simulink model "IndustrialMicrogrid"  (R2023a)
settings: Solver=FixedStepDiscrete  StartTime=0.0  StopTime=10  FixedStep=Ts  RelTol=1e-3
PostLoadFcn:
  | IndustrialMicrogridInputData
  | GfmGridFormingConverterInputParameters
model workspace (MAT data in the model file):
  caseNum = 2
undefined symbols (not defined in the file): base, BESS, DiscIntNeverNeededParam, grid, Grid, gridInverter, machine, microgrid, PV, PVInverter, PVTransformer, scrFactorRg, scrFactorXg, transformer, Ts
libraries: ee_lib x112, eeGeneralControl x104, nesl_utility_internal x64, simulink x56, nesl_utility x37, fl_lib x29, slpidlib x13, eeTransforms x11, eeTotalHarmonicDistorsion x8, eeRmsMeasurement x4, eeSinusoidalMeasurement x4, simulink_extras x2
(part 8 of 14)

== system IndustrialMicrogrid/MG2 Primary Substation/Microgrid Controller 2/Planned Island/Control for Zero Powerflow1 ==
  Bus Element In{,1..4} (5 alike) : Inport  PortName=ControlRoom  Element=PlannedIslandCmd2
  In Bus Element7 : Inport  Port=2  PortName=mPCCPLL2  Element=PCC2.mPCC2.activepower
  In Bus Element1 : Inport  Port=2  PortName=mPCCPLL2  Element=PCC2.mPCC2.reactivepower
  Logical Operator : Logic  AllPortsSameDT=off  OutDataTypeStr=boolean
  PID Frequency : slpidlib/PID Controller  Controller=PI  Form=Parallel  TimeDomain=Discrete-time  UseExternalTs=off  SampleTime=2*Ts  IntegratorMethod=Forward Euler  FilterMethod=Forward Euler  ControllerParametersSource=internal  P=KpPPlannedIsland  I=KiPPlannedIsland  UseKiTs=off  D=0  N=100  UseFilter=on  TunerSelectOption=Frequency Response Based  InitialConditionSource=internal  InitialConditionForIntegrator=0  InitialConditionForFilter=0  DifferentiatorICPrevScaledInput=0  ExternalReset=none  TrackingMode=off  Kt=1  LimitOutput=off  SatLimitsSource=internal  UpperSaturationLimit=0.05  LowerSaturationLimit=-0.05  LinearizeAsGain=on  AntiWindupMode=clamping  Kb=1  LimitIntegrator=off  UpperIntegratorSaturationLimit=inf  LowerIntegratorSaturationLimit=-inf  POutMin=[]  POutMax=[]  IOutMin=[]  IOutMax=[]  DOutMin=[]  DOutMax=[]  NOutMin=[]  NOutMax=[]  SumOutMin=[]  SumOutMax=[]  SaturationOutMin=[]  SaturationOutMax=[]  PParamMin=[]  PParamMax=[]  IParamMin=[]  IParamMax=[]  DParamMin=[]  DParamMax=[]  NParamMin=[]  NParamMax=[]  KbParamMin=[]  KbParamMax=[]  KtParamMin=[]  KtParamMax=[]  KbOutMin=[]  KbOutMax=[]  KtOutMin=[]  KtOutMax=[]  IntegratorOutMin=[]  IntegratorOutMax=[]  FilterOutMin=[]  FilterOutMax=[]  SumI1OutMin=[]  SumI1OutMax=[]  SumI2OutMin=[]  SumI2OutMax=[]  SumI3OutMin=[]  SumI3OutMax=[]  SumI4OutMin=[]  SumI4OutMax=[]  SumDOutMin=[]  SumDOutMax=[]  DifferentiatorOutMin=[]  DifferentiatorOutMax=[]  FilterDiffOutCoefMin=[]  FilterDiffOutCoefMax=[]  ReciprocalOutMin=[]  ReciprocalOutMax=[]  SumDenOutMin=[]  SumDenOutMax=[]  SumNumOutMin=[]  SumNumOutMax=[]  DivideOutMin=[]  DivideOutMax=[]  UdiffTsProdOutMin=[]  UdiffTsProdOutMax=[]  NTsProdOutMin=[]  NTsProdOutMax=[]  UintegralTsProdOutMin=[]  UintegralTsProdOutMax=[]  UngainTsProdOutMin=[]  UngainTsProdOutMax=[]  ClampingZeroOutDataTypeStr=Inherit: Inherit via back propagation  ClampingZeroOutMin=[]  ClampingZeroOutMax=[]  FilterDenConstantOutDataTypeStr=Inherit: Inherit via back propagation  FilterDenConstantOutMin=[]  FilterDenConstantOutMax=[]  PCopyOutDataTypeStr=Inherit: Inherit via back propagation  PCopyOutMin=[]  PCopyOutMax=[]  NCopyOutDataTypeStr=Inherit: Inherit via back propagation  NCopyOutMin=[]  NCopyOutMax=[]  IntegratorContinuousStateAttributes=''  IntegratorStateMustResolveToSignalObject=off  IntegratorRTWStateStorageClass=Auto  FilterContinuousStateAttributes=''  FilterStateMustResolveToSignalObject=off  FilterRTWStateStorageClass=Auto  ParallelPVariant=InternalParameters  IdealPVariant=Disabled  IVariant=InternalParameters  DVariant=Disabled  IntegratorVariant=Discrete  SatVariant=Disabled  AWVariant=Passthrough  PCopyVariant=Disabled  TRVariant=Disabled  FdbkBlocksVariant=Forward  IdealPFdbkVariant=Disabled  SatFdbkVariant=Disabled  DerivativeFilterVariant=Disabled  NVariant=Disabled  NCopyVariant=Disabled_SignalSpec  FilterICVariant=Disabled  IntegratorICVariant=InternalICs  ExternalResetVariant=Disabled  TRSumVariant=Passthrough  SumFdbkVariant=Disabled  SumVariant=Sum_PI  TsampFilterVariant=InternalTs  TsampNgainVariant=Passthrough  TsampIntegralVariant=Disabled_SignalSpec  ExternalSaturationOutDataTypeStr=Inherit: Same as second input
  PID voltage : slpidlib/PID Controller  Controller=PI  Form=Parallel  TimeDomain=Discrete-time  UseExternalTs=off  SampleTime=2*Ts  IntegratorMethod=Forward Euler  FilterMethod=Forward Euler  ControllerParametersSource=internal  P=KpQPlannedIsland  I=KiQPlannedIsland  UseKiTs=off  D=0  N=100  UseFilter=on  TunerSelectOption=Frequency Response Based  InitialConditionSource=internal  InitialConditionForIntegrator=0  InitialConditionForFilter=0  DifferentiatorICPrevScaledInput=0  ExternalReset=none  TrackingMode=off  Kt=1  LimitOutput=off  SatLimitsSource=internal  UpperSaturationLimit=0.05  LowerSaturationLimit=-0.05  LinearizeAsGain=on  AntiWindupMode=clamping  Kb=1  LimitIntegrator=off  UpperIntegratorSaturationLimit=inf  LowerIntegratorSaturationLimit=-inf  POutMin=[]  POutMax=[]  IOutMin=[]  IOutMax=[]  DOutMin=[]  DOutMax=[]  NOutMin=[]  NOutMax=[]  SumOutMin=[]  SumOutMax=[]  SaturationOutMin=[]  SaturationOutMax=[]  PParamMin=[]  PParamMax=[]  IParamMin=[]  IParamMax=[]  DParamMin=[]  DParamMax=[]  NParamMin=[]  NParamMax=[]  KbParamMin=[]  KbParamMax=[]  KtParamMin=[]  KtParamMax=[]  KbOutMin=[]  KbOutMax=[]  KtOutMin=[]  KtOutMax=[]  IntegratorOutMin=[]  IntegratorOutMax=[]  FilterOutMin=[]  FilterOutMax=[]  SumI1OutMin=[]  SumI1OutMax=[]  SumI2OutMin=[]  SumI2OutMax=[]  SumI3OutMin=[]  SumI3OutMax=[]  SumI4OutMin=[]  SumI4OutMax=[]  SumDOutMin=[]  SumDOutMax=[]  DifferentiatorOutMin=[]  DifferentiatorOutMax=[]  FilterDiffOutCoefMin=[]  FilterDiffOutCoefMax=[]  ReciprocalOutMin=[]  ReciprocalOutMax=[]  SumDenOutMin=[]  SumDenOutMax=[]  SumNumOutMin=[]  SumNumOutMax=[]  DivideOutMin=[]  DivideOutMax=[]  UdiffTsProdOutMin=[]  UdiffTsProdOutMax=[]  NTsProdOutMin=[]  NTsProdOutMax=[]  UintegralTsProdOutMin=[]  UintegralTsProdOutMax=[]  UngainTsProdOutMin=[]  UngainTsProdOutMax=[]  ClampingZeroOutDataTypeStr=Inherit: Inherit via back propagation  ClampingZeroOutMin=[]  ClampingZeroOutMax=[]  FilterDenConstantOutDataTypeStr=Inherit: Inherit via back propagation  FilterDenConstantOutMin=[]  FilterDenConstantOutMax=[]  PCopyOutDataTypeStr=Inherit: Inherit via back propagation  PCopyOutMin=[]  PCopyOutMax=[]  NCopyOutDataTypeStr=Inherit: Inherit via back propagation  NCopyOutMin=[]  NCopyOutMax=[]  IntegratorContinuousStateAttributes=''  IntegratorStateMustResolveToSignalObject=off  IntegratorRTWStateStorageClass=Auto  FilterContinuousStateAttributes=''  FilterStateMustResolveToSignalObject=off  FilterRTWStateStorageClass=Auto  ParallelPVariant=InternalParameters  IdealPVariant=Disabled  IVariant=InternalParameters  DVariant=Disabled  IntegratorVariant=Discrete  SatVariant=Disabled  AWVariant=Passthrough  PCopyVariant=Disabled  TRVariant=Disabled  FdbkBlocksVariant=Forward  IdealPFdbkVariant=Disabled  SatFdbkVariant=Disabled  DerivativeFilterVariant=Disabled  NVariant=Disabled  NCopyVariant=Disabled_SignalSpec  FilterICVariant=Disabled  IntegratorICVariant=InternalICs  ExternalResetVariant=Disabled  TRSumVariant=Passthrough  SumFdbkVariant=Disabled  SumVariant=Sum_PI  TsampFilterVariant=InternalTs  TsampNgainVariant=Passthrough  TsampIntegralVariant=Disabled_SignalSpec  ExternalSaturationOutDataTypeStr=Inherit: Same as second input
  Planned Island Time Delay : Subsystem
  Product{,1..3} (4 alike) : Product
  Subsystem : Subsystem
  Subsystem1 : Subsystem
  Bus Element Out : Outport  PortName=MGController2  Element=plannedisland
  Bus Element Out1 : Outport  PortName=MGController2  Element=plannedislandP
  Bus Element Out2 : Outport  PortName=MGController2  Element=plannedislandQ
  Bus Element Out4 : Outport  PortName=MGController2  Element=activepowererror
  Bus Element Out6 : Outport  PortName=MGController2  Element=reactivepowerrror
  wires:
  Logical Operator/1 -> Planned Island Time Delay/1(In1)
  Planned Island Time Delay/1(MGController) -> Bus Element Out/1
  Bus Element In3/1 -> Planned Island Time Delay/2(In2)
  PID voltage/1 -> Bus Element Out2/1  "REACTIVE POWER"
  Bus Element In2/1 -> Product2/2
  Bus Element In/1 -> Product1/2
  Product2/1 -> Subsystem1/1(REACTIVEPOWER ERROR), PID voltage/1, Bus Element Out6/1  "REACTIVEPOWER ERROR"
  Product1/1 -> PID Frequency/1, Bus Element Out4/1, Subsystem/1(AVTIVE POWER ERROR)  "AVTIVE POWER ERROR"
  PID Frequency/1 -> Bus Element Out1/1  "ACTIVE POWER"
  In Bus Element1/1 -> Product2/1
  In Bus Element7/1 -> Product1/1
  Bus Element In1/1 -> Product/1
  Product/1 -> Logical Operator/1
  Product3/1 -> Logical Operator/2
  Bus Element In4/1 -> Product3/1
  Subsystem/1(Out1) -> Product/2
  Subsystem1/1(Out1) -> Product3/2

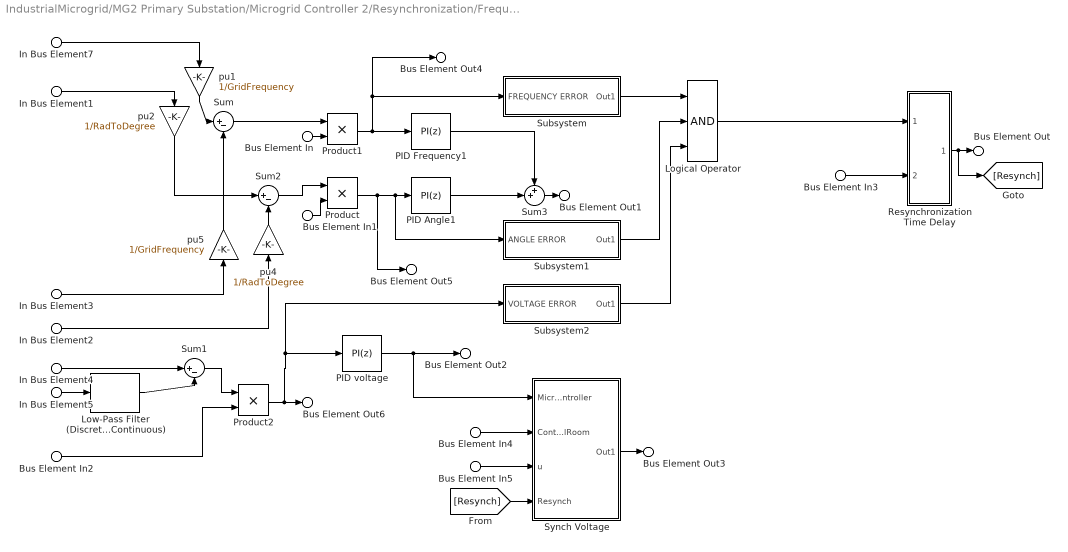
== system IndustrialMicrogrid/MG2 Primary Substation/Microgrid Controller 2/Resynchronization/Frequency and voltage matching ==
  Bus Element In5 : Inport  PortName=BESS2  Element=reactive power
  Bus Element In{,1..4} (5 alike) : Inport  Port=2  PortName=ControlRoom  Element=ResynchCmd2
  In Bus Element7 : Inport  Port=3  PortName=mPCCPLL2  Element=Grid2.frequency
  In Bus Element1 : Inport  Port=3  PortName=mPCCPLL2  Element=Grid2.angle
  In Bus Element4 : Inport  Port=3  PortName=mPCCPLL2  Element=Grid2.voltage
  In Bus Element3 : Inport  Port=3  PortName=mPCCPLL2  Element=Island2.frequency
  In Bus Element2 : Inport  Port=3  PortName=mPCCPLL2  Element=Island2.angle
  In Bus Element5 : Inport  Port=3  PortName=mPCCPLL2  Element=Island2.voltage
  Logical Operator : Logic  Inputs=3  AllPortsSameDT=off  OutDataTypeStr=boolean
  Low-Pass Filter (Discrete or Continuous) : eeGeneralControl/Low-Pass Filter (Discrete or Continuous)  K=1  T=0.04  B=inf  A=-inf  init_option=Inherited from block input  x0=0  Ts=-1
  PID Angle1 : slpidlib/PID Controller  Controller=PI  Form=Parallel  TimeDomain=Discrete-time  UseExternalTs=off  SampleTime=2*Ts  IntegratorMethod=Forward Euler  FilterMethod=Forward Euler  ControllerParametersSource=internal  P=KpAngResynch  I=KiAngResynch  UseKiTs=off  D=0  N=100  UseFilter=on  TunerSelectOption=Frequency Response Based  InitialConditionSource=internal  InitialConditionForIntegrator=0  InitialConditionForFilter=0  DifferentiatorICPrevScaledInput=0  ExternalReset=none  TrackingMode=off  Kt=1  LimitOutput=off  SatLimitsSource=internal  UpperSaturationLimit=0.05  LowerSaturationLimit=-0.05  LinearizeAsGain=on  AntiWindupMode=clamping  Kb=1  LimitIntegrator=off  UpperIntegratorSaturationLimit=inf  LowerIntegratorSaturationLimit=-inf  POutMin=[]  POutMax=[]  IOutMin=[]  IOutMax=[]  DOutMin=[]  DOutMax=[]  NOutMin=[]  NOutMax=[]  SumOutMin=[]  SumOutMax=[]  SaturationOutMin=[]  SaturationOutMax=[]  PParamMin=[]  PParamMax=[]  IParamMin=[]  IParamMax=[]  DParamMin=[]  DParamMax=[]  NParamMin=[]  NParamMax=[]  KbParamMin=[]  KbParamMax=[]  KtParamMin=[]  KtParamMax=[]  KbOutMin=[]  KbOutMax=[]  KtOutMin=[]  KtOutMax=[]  IntegratorOutMin=[]  IntegratorOutMax=[]  FilterOutMin=[]  FilterOutMax=[]  SumI1OutMin=[]  SumI1OutMax=[]  SumI2OutMin=[]  SumI2OutMax=[]  SumI3OutMin=[]  SumI3OutMax=[]  SumI4OutMin=[]  SumI4OutMax=[]  SumDOutMin=[]  SumDOutMax=[]  DifferentiatorOutMin=[]  DifferentiatorOutMax=[]  FilterDiffOutCoefMin=[]  FilterDiffOutCoefMax=[]  ReciprocalOutMin=[]  ReciprocalOutMax=[]  SumDenOutMin=[]  SumDenOutMax=[]  SumNumOutMin=[]  SumNumOutMax=[]  DivideOutMin=[]  DivideOutMax=[]  UdiffTsProdOutMin=[]  UdiffTsProdOutMax=[]  NTsProdOutMin=[]  NTsProdOutMax=[]  UintegralTsProdOutMin=[]  UintegralTsProdOutMax=[]  UngainTsProdOutMin=[]  UngainTsProdOutMax=[]  ClampingZeroOutDataTypeStr=Inherit: Inherit via back propagation  ClampingZeroOutMin=[]  ClampingZeroOutMax=[]  FilterDenConstantOutDataTypeStr=Inherit: Inherit via back propagation  FilterDenConstantOutMin=[]  FilterDenConstantOutMax=[]  PCopyOutDataTypeStr=Inherit: Inherit via back propagation  PCopyOutMin=[]  PCopyOutMax=[]  NCopyOutDataTypeStr=Inherit: Inherit via back propagation  NCopyOutMin=[]  NCopyOutMax=[]  IntegratorContinuousStateAttributes=''  IntegratorStateMustResolveToSignalObject=off  IntegratorRTWStateStorageClass=Auto  FilterContinuousStateAttributes=''  FilterStateMustResolveToSignalObject=off  FilterRTWStateStorageClass=Auto  ParallelPVariant=InternalParameters  IdealPVariant=Disabled  IVariant=InternalParameters  DVariant=Disabled  IntegratorVariant=Discrete  SatVariant=Disabled  AWVariant=Passthrough  PCopyVariant=Disabled  TRVariant=Disabled  FdbkBlocksVariant=Forward  IdealPFdbkVariant=Disabled  SatFdbkVariant=Disabled  DerivativeFilterVariant=Disabled  NVariant=Disabled  NCopyVariant=Disabled_SignalSpec  FilterICVariant=Disabled  IntegratorICVariant=InternalICs  ExternalResetVariant=Disabled  TRSumVariant=Passthrough  SumFdbkVariant=Disabled  SumVariant=Sum_PI  TsampFilterVariant=InternalTs  TsampNgainVariant=Passthrough  TsampIntegralVariant=Disabled_SignalSpec  ExternalSaturationOutDataTypeStr=Inherit: Same as second input
  PID Frequency1 : slpidlib/PID Controller  Controller=PI  Form=Parallel  TimeDomain=Discrete-time  UseExternalTs=off  SampleTime=2*Ts  IntegratorMethod=Forward Euler  FilterMethod=Forward Euler  ControllerParametersSource=internal  P=KpFreResynch  I=KiFreResynch  UseKiTs=off  D=0  N=100  UseFilter=on  TunerSelectOption=Frequency Response Based  InitialConditionSource=internal  InitialConditionForIntegrator=0  InitialConditionForFilter=0  DifferentiatorICPrevScaledInput=0  ExternalReset=none  TrackingMode=off  Kt=1  LimitOutput=off  SatLimitsSource=internal  UpperSaturationLimit=0.05  LowerSaturationLimit=-0.05  LinearizeAsGain=on  AntiWindupMode=clamping  Kb=1  LimitIntegrator=off  UpperIntegratorSaturationLimit=inf  LowerIntegratorSaturationLimit=-inf  POutMin=[]  POutMax=[]  IOutMin=[]  IOutMax=[]  DOutMin=[]  DOutMax=[]  NOutMin=[]  NOutMax=[]  SumOutMin=[]  SumOutMax=[]  SaturationOutMin=[]  SaturationOutMax=[]  PParamMin=[]  PParamMax=[]  IParamMin=[]  IParamMax=[]  DParamMin=[]  DParamMax=[]  NParamMin=[]  NParamMax=[]  KbParamMin=[]  KbParamMax=[]  KtParamMin=[]  KtParamMax=[]  KbOutMin=[]  KbOutMax=[]  KtOutMin=[]  KtOutMax=[]  IntegratorOutMin=[]  IntegratorOutMax=[]  FilterOutMin=[]  FilterOutMax=[]  SumI1OutMin=[]  SumI1OutMax=[]  SumI2OutMin=[]  SumI2OutMax=[]  SumI3OutMin=[]  SumI3OutMax=[]  SumI4OutMin=[]  SumI4OutMax=[]  SumDOutMin=[]  SumDOutMax=[]  DifferentiatorOutMin=[]  DifferentiatorOutMax=[]  FilterDiffOutCoefMin=[]  FilterDiffOutCoefMax=[]  ReciprocalOutMin=[]  ReciprocalOutMax=[]  SumDenOutMin=[]  SumDenOutMax=[]  SumNumOutMin=[]  SumNumOutMax=[]  DivideOutMin=[]  DivideOutMax=[]  UdiffTsProdOutMin=[]  UdiffTsProdOutMax=[]  NTsProdOutMin=[]  NTsProdOutMax=[]  UintegralTsProdOutMin=[]  UintegralTsProdOutMax=[]  UngainTsProdOutMin=[]  UngainTsProdOutMax=[]  ClampingZeroOutDataTypeStr=Inherit: Inherit via back propagation  ClampingZeroOutMin=[]  ClampingZeroOutMax=[]  FilterDenConstantOutDataTypeStr=Inherit: Inherit via back propagation  FilterDenConstantOutMin=[]  FilterDenConstantOutMax=[]  PCopyOutDataTypeStr=Inherit: Inherit via back propagation  PCopyOutMin=[]  PCopyOutMax=[]  NCopyOutDataTypeStr=Inherit: Inherit via back propagation  NCopyOutMin=[]  NCopyOutMax=[]  IntegratorContinuousStateAttributes=''  IntegratorStateMustResolveToSignalObject=off  IntegratorRTWStateStorageClass=Auto  FilterContinuousStateAttributes=''  FilterStateMustResolveToSignalObject=off  FilterRTWStateStorageClass=Auto  ParallelPVariant=InternalParameters  IdealPVariant=Disabled  IVariant=InternalParameters  DVariant=Disabled  IntegratorVariant=Discrete  SatVariant=Disabled  AWVariant=Passthrough  PCopyVariant=Disabled  TRVariant=Disabled  FdbkBlocksVariant=Forward  IdealPFdbkVariant=Disabled  SatFdbkVariant=Disabled  DerivativeFilterVariant=Disabled  NVariant=Disabled  NCopyVariant=Disabled_SignalSpec  FilterICVariant=Disabled  IntegratorICVariant=InternalICs  ExternalResetVariant=Disabled  TRSumVariant=Passthrough  SumFdbkVariant=Disabled  SumVariant=Sum_PI  TsampFilterVariant=InternalTs  TsampNgainVariant=Passthrough  TsampIntegralVariant=Disabled_SignalSpec  ExternalSaturationOutDataTypeStr=Inherit: Same as second input
  PID voltage : slpidlib/PID Controller  Controller=PI  Form=Parallel  TimeDomain=Discrete-time  UseExternalTs=off  SampleTime=2*Ts  IntegratorMethod=Forward Euler  FilterMethod=Forward Euler  ControllerParametersSource=internal  P=KpVolResynch  I=KiVolResynch  UseKiTs=off  D=0  N=100  UseFilter=on  TunerSelectOption=Frequency Response Based  InitialConditionSource=internal  InitialConditionForIntegrator=1  InitialConditionForFilter=0  DifferentiatorICPrevScaledInput=0  ExternalReset=none  TrackingMode=off  Kt=1  LimitOutput=off  SatLimitsSource=internal  UpperSaturationLimit=0.05  LowerSaturationLimit=-0.05  LinearizeAsGain=on  AntiWindupMode=clamping  Kb=1  LimitIntegrator=off  UpperIntegratorSaturationLimit=inf  LowerIntegratorSaturationLimit=-inf  POutMin=[]  POutMax=[]  IOutMin=[]  IOutMax=[]  DOutMin=[]  DOutMax=[]  NOutMin=[]  NOutMax=[]  SumOutMin=[]  SumOutMax=[]  SaturationOutMin=[]  SaturationOutMax=[]  PParamMin=[]  PParamMax=[]  IParamMin=[]  IParamMax=[]  DParamMin=[]  DParamMax=[]  NParamMin=[]  NParamMax=[]  KbParamMin=[]  KbParamMax=[]  KtParamMin=[]  KtParamMax=[]  KbOutMin=[]  KbOutMax=[]  KtOutMin=[]  KtOutMax=[]  IntegratorOutMin=[]  IntegratorOutMax=[]  FilterOutMin=[]  FilterOutMax=[]  SumI1OutMin=[]  SumI1OutMax=[]  SumI2OutMin=[]  SumI2OutMax=[]  SumI3OutMin=[]  SumI3OutMax=[]  SumI4OutMin=[]  SumI4OutMax=[]  SumDOutMin=[]  SumDOutMax=[]  DifferentiatorOutMin=[]  DifferentiatorOutMax=[]  FilterDiffOutCoefMin=[]  FilterDiffOutCoefMax=[]  ReciprocalOutMin=[]  ReciprocalOutMax=[]  SumDenOutMin=[]  SumDenOutMax=[]  SumNumOutMin=[]  SumNumOutMax=[]  DivideOutMin=[]  DivideOutMax=[]  UdiffTsProdOutMin=[]  UdiffTsProdOutMax=[]  NTsProdOutMin=[]  NTsProdOutMax=[]  UintegralTsProdOutMin=[]  UintegralTsProdOutMax=[]  UngainTsProdOutMin=[]  UngainTsProdOutMax=[]  ClampingZeroOutDataTypeStr=Inherit: Inherit via back propagation  ClampingZeroOutMin=[]  ClampingZeroOutMax=[]  FilterDenConstantOutDataTypeStr=Inherit: Inherit via back propagation  FilterDenConstantOutMin=[]  FilterDenConstantOutMax=[]  PCopyOutDataTypeStr=Inherit: Inherit via back propagation  PCopyOutMin=[]  PCopyOutMax=[]  NCopyOutDataTypeStr=Inherit: Inherit via back propagation  NCopyOutMin=[]  NCopyOutMax=[]  IntegratorContinuousStateAttributes=''  IntegratorStateMustResolveToSignalObject=off  IntegratorRTWStateStorageClass=Auto  FilterContinuousStateAttributes=''  FilterStateMustResolveToSignalObject=off  FilterRTWStateStorageClass=Auto  ParallelPVariant=InternalParameters  IdealPVariant=Disabled  IVariant=InternalParameters  DVariant=Disabled  IntegratorVariant=Discrete  SatVariant=Disabled  AWVariant=Passthrough  PCopyVariant=Disabled  TRVariant=Disabled  FdbkBlocksVariant=Forward  IdealPFdbkVariant=Disabled  SatFdbkVariant=Disabled  DerivativeFilterVariant=Disabled  NVariant=Disabled  NCopyVariant=Disabled_SignalSpec  FilterICVariant=Disabled  IntegratorICVariant=InternalICs  ExternalResetVariant=Disabled  TRSumVariant=Passthrough  SumFdbkVariant=Disabled  SumVariant=Sum_PI  TsampFilterVariant=InternalTs  TsampNgainVariant=Passthrough  TsampIntegralVariant=Disabled_SignalSpec  ExternalSaturationOutDataTypeStr=Inherit: Same as second input
  Product : Product
  Product1 : Product
  Product2 : Product
  Resynchronization Time Delay : Subsystem
  Subsystem : Subsystem
  Subsystem1 : Subsystem
  Subsystem2 : Subsystem
  Sum : Sum  Inputs=|+-
  Sum1 : Sum  Inputs=|+-
  Sum2 : Sum  Inputs=|+-
  Sum3 : Sum  Inputs=++|
  Synch Voltage : Subsystem
  pu1 : Gain  Gain=1/GridFrequency
  pu2 : Gain  Gain=1/RadToDegree
  pu4 : Gain  Gain=1/RadToDegree
  pu5 : Gain  Gain=1/GridFrequency
  Bus Element Out : Outport  PortName=MGController2  Element=resynch
  Bus Element Out1 : Outport  PortName=MGController2  Element=synchfrequency
  Bus Element Out2 : Outport  PortName=MGController2  Element=synchvoltage
  Bus Element Out3 : Outport  PortName=MGController2  Element=synchvoltagedpr
  Bus Element Out4 : Outport  PortName=MGController2  Element=frequencyerror
  Bus Element Out5 : Outport  PortName=MGController2  Element=phaseerror
  Bus Element Out6 : Outport  PortName=MGController2  Element=voltagemagerror
  wires:
  Sum/1 -> Product1/1
  pu1/1 -> Sum/1
  pu4/1 -> Sum2/2
  pu2/1 -> Sum2/1
  pu5/1 -> Sum/2
  In Bus Element2/1 -> pu4/1
  In Bus Element3/1 -> pu5/1
  Sum1/1 -> Product2/1
  Subsystem/1(Out1) -> Logical Operator/1
  Subsystem1/1(Out1) -> Logical Operator/2
  Subsystem2/1(Out1) -> Logical Operator/3
  Sum3/1 -> Bus Element Out1/1
  PID Frequency1/1 -> Sum3/1
  PID Angle1/1 -> Sum3/2
  Sum2/1 -> Product/1
  Product/1 -> Bus Element Out5/1, Subsystem1/1(ANGLE ERROR), PID Angle1/1
  Product1/1 -> Bus Element Out4/1, Subsystem/1(FREQUENCY ERROR), PID Frequency1/1
  Product2/1 -> Subsystem2/1(VOLTAGE ERROR), PID voltage/1, Bus Element Out6/1
  Bus Element In/1 -> Product1/2
  Bus Element In1/1 -> Product/2
  Bus Element In2/1 -> Product2/2
  In Bus Element7/1 -> pu1/1
  In Bus Element1/1 -> pu2/1
  In Bus Element4/1 -> Sum1/1
  In Bus Element5/1 -> Low-Pass Filter (Discrete or Continuous)/1
  PID voltage/1 -> Bus Element Out2/1, Synch Voltage/1(MicrogridController)
  Bus Element In3/1 -> Resynchronization Time Delay/2(In2)
  Resynchronization Time Delay/1(MGController) -> [Resynch], Bus Element Out/1
  Logical Operator/1 -> Resynchronization Time Delay/1(In1)
  Bus Element In4/1 -> Synch Voltage/2(ControlRoom)
  Bus Element In5/1 -> Synch Voltage/3(u)
  Synch Voltage/1(Out1) -> Bus Element Out3/1
  [Resynch] -> Synch Voltage/4(Resynch)
  Low-Pass Filter (Discrete or Continuous)/1 -> Sum1/2

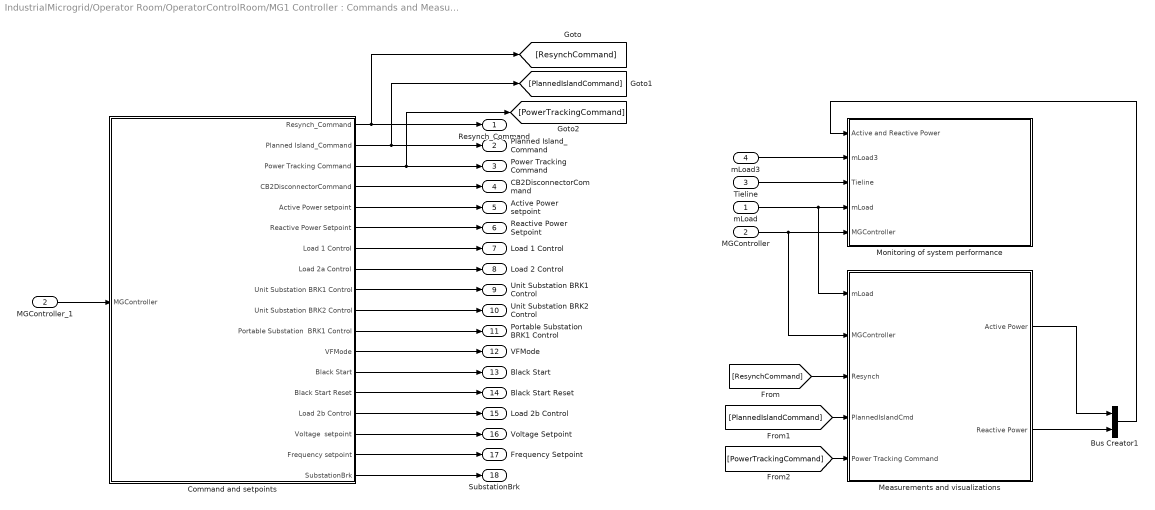
== system IndustrialMicrogrid/Operator Room/OperatorControlRoom/MG1 Controller : Commands and Measurements/Microgrid Controller 1 : Commands and Measurements ==
  mLoad : Inport
  MGController : Inport  Port=2
  Tieline : Inport  Port=3
  mLoad3 : Inport  Port=4
  Bus Creator1 : BusCreator  Inputs=2
  Command and setpoints : Subsystem
  MGController_1 : InportShadow  Port=2
  "Measurements and visualizations " : Subsystem
  Monitoring of system performance : Subsystem
  Resynch_Command : Outport
  Planned Island_Command : Outport  Port=2
  Power Tracking Command : Outport  Port=3
  CB2DisconnectorCommand : Outport  Port=4
  Active Power setpoint : Outport  Port=5
  Reactive Power Setpoint : Outport  Port=6
  Load 1 Control : Outport  Port=7
  Load 2 Control : Outport  Port=8
  Unit Substation BRK1 Control : Outport  Port=9
  Unit Substation BRK2 Control : Outport  Port=10
  Portable Substation  BRK1 Control : Outport  Port=11
  VFMode : Outport  Port=12
  Black Start : Outport  Port=13
  Black Start Reset : Outport  Port=14
  Load 2b Control : Outport  Port=15
  Voltage Setpoint : Outport  Port=16
  Frequency Setpoint : Outport  Port=17
  SubstationBrk : Outport  Port=18
  wires:
  mLoad/1 -> "Measurements and visualizations "/1(mLoad), Monitoring of system performance/4(mLoad)
  [PlannedIslandCommand] -> "Measurements and visualizations "/4(PlannedIslandCmd)
  Command and setpoints/2(Planned Island_Command) -> Planned Island_Command/1, [PlannedIslandCommand]
  Command and setpoints/3(Power Tracking Command) -> Power Tracking Command/1, [PowerTrackingCommand]
  Command and setpoints/1(Resynch_Command) -> Resynch_Command/1, [ResynchCommand]
  Command and setpoints/4(CB2DisconnectorCommand) -> CB2DisconnectorCommand/1
  MGController/1 -> "Measurements and visualizations "/2(MGController), Monitoring of system performance/5(MGController)
  MGController_1/1 -> Command and setpoints/1(MGController)
  [ResynchCommand] -> "Measurements and visualizations "/3(Resynch)
  [PowerTrackingCommand] -> "Measurements and visualizations "/5(Power Tracking Command)
  Command and setpoints/5(Active Power setpoint) -> Active Power setpoint/1
  Command and setpoints/6(Reactive Power Setpoint) -> Reactive Power Setpoint/1
  Command and setpoints/10(Unit Substation BRK2 Control) -> Unit Substation BRK2 Control/1
  Command and setpoints/8(Load 2a Control) -> Load 2 Control/1
  Command and setpoints/9(Unit Substation BRK1 Control) -> Unit Substation BRK1 Control/1
  Command and setpoints/7(Load 1 Control) -> Load 1 Control/1
  Command and setpoints/11(Portable Substation  BRK1 Control) -> Portable Substation  BRK1 Control/1
  Command and setpoints/12(VFMode) -> VFMode/1
  Command and setpoints/14(Black Start Reset) -> Black Start Reset/1
  Command and setpoints/13(Black Start) -> Black Start/1
  Command and setpoints/15(Load 2b Control) -> Load 2b Control/1
  Command and setpoints/16(Voltage  setpoint) -> Voltage Setpoint/1
  Command and setpoints/17(Frequency setpoint) -> Frequency Setpoint/1
  Command and setpoints/18(SubstationBrk) -> SubstationBrk/1
  "Measurements and visualizations "/2(Reactive Power) -> Bus Creator1/2
  "Measurements and visualizations "/1(Active Power) -> Bus Creator1/1
  Bus Creator1/1 -> Monitoring of system performance/1(Active and Reactive Power)
  Tieline/1 -> Monitoring of system performance/3(Tieline)
  mLoad3/1 -> Monitoring of system performance/2(mLoad3)

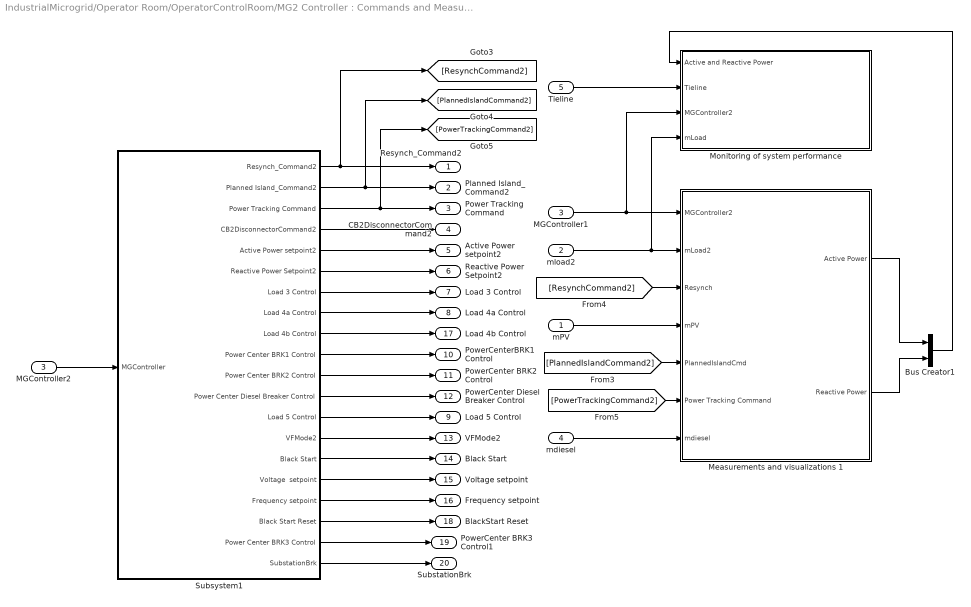
== system IndustrialMicrogrid/Operator Room/OperatorControlRoom/MG2 Controller : Commands and Measurements/Microgrid Controller 2 : Commands and Measurements ==
  mPV : Inport
  mload2 : Inport  Port=2
  MGController2 : Inport  Port=3
  mdiesel : Inport  Port=4
  Tieline : Inport  Port=5
  Bus Creator1 : BusCreator  Inputs=2
  MGController1 : InportShadow  Port=3
  Measurements and visualizations 1 : Subsystem
  Monitoring of system performance : Subsystem
  Subsystem1 : Subsystem
  Resynch_Command2 : Outport
  Planned Island_Command2 : Outport  Port=2
  Power Tracking Command : Outport  Port=3
  CB2DisconnectorCommand2 : Outport  Port=4
  Active Power setpoint2 : Outport  Port=5
  Reactive Power Setpoint2 : Outport  Port=6
  Load 3 Control : Outport  Port=7
  Load 4a Control : Outport  Port=8
  Load 5 Control : Outport  Port=9
  PowerCenterBRK1 Control : Outport  Port=10
  PowerCenter BRK2 Control : Outport  Port=11
  PowerCenter Diesel Breaker Control : Outport  Port=12
  VFMode2 : Outport  Port=13
  Black Start : Outport  Port=14
  Voltage setpoint : Outport  Port=15
  Frequency setpoint : Outport  Port=16
  Load 4b Control : Outport  Port=17
  BlackStart Reset : Outport  Port=18
  PowerCenter BRK3 Control1 : Outport  Port=19
  SubstationBrk : Outport  Port=20
  wires:
  Subsystem1/2(Planned Island_Command2) -> Planned Island_Command2/1, [PlannedIslandCommand2]
  [PlannedIslandCommand2] -> Measurements and visualizations 1/5(PlannedIslandCmd)
  Subsystem1/11(Power Center BRK2 Control) -> PowerCenter BRK2 Control/1
  MGController2/1 -> Subsystem1/1(MGController)
  Subsystem1/1(Resynch_Command2) -> Resynch_Command2/1, [ResynchCommand2]
  mload2/1 -> Monitoring of system performance/4(mLoad), Measurements and visualizations 1/2(mLoad2)
  [ResynchCommand2] -> Measurements and visualizations 1/3(Resynch)
  mPV/1 -> Measurements and visualizations 1/4(mPV)
  Subsystem1/3(Power Tracking Command) -> Power Tracking Command/1, [PowerTrackingCommand2]
  Subsystem1/6(Reactive Power Setpoint2) -> Reactive Power Setpoint2/1
  mdiesel/1 -> Measurements and visualizations 1/7(mdiesel)
  [PowerTrackingCommand2] -> Measurements and visualizations 1/6(Power Tracking Command)
  Subsystem1/4(CB2DisconnectorCommand2) -> CB2DisconnectorCommand2/1
  Subsystem1/10(Power Center BRK1 Control) -> PowerCenterBRK1 Control/1
  Subsystem1/5(Active Power setpoint2) -> Active Power setpoint2/1
  Subsystem1/8(Load 4a Control) -> Load 4a Control/1
  Subsystem1/12(Power Center Diesel Breaker Control) -> PowerCenter Diesel Breaker Control/1
  Subsystem1/7(Load 3 Control) -> Load 3 Control/1
  Subsystem1/13(Load 5 Control) -> Load 5 Control/1
  Subsystem1/14(VFMode2) -> VFMode2/1
  Subsystem1/15(Black Start) -> Black Start/1
  Subsystem1/16(Voltage  setpoint) -> Voltage setpoint/1
  Subsystem1/17(Frequency setpoint) -> Frequency setpoint/1
  Subsystem1/9(Load 4b Control) -> Load 4b Control/1
  Subsystem1/18(Black Start Reset) -> BlackStart Reset/1
  Subsystem1/19(Power Center BRK3 Control) -> PowerCenter BRK3 Control1/1
  Subsystem1/20(SubstationBrk) -> SubstationBrk/1
  MGController1/1 -> Measurements and visualizations 1/1(MGController2), Monitoring of system performance/3(MGController2)
  Measurements and visualizations 1/1(Active Power) -> Bus Creator1/1
  Measurements and visualizations 1/2(Reactive Power) -> Bus Creator1/2
  Bus Creator1/1 -> Monitoring of system performance/1(Active and Reactive Power)
  Tieline/1 -> Monitoring of system performance/2(Tieline)

== system IndustrialMicrogrid/MG1 Primary Substation/BESS and Controller/BESS/Grid-Forming Converter Control/Current Limiting ==
  In Bus Element : Inport  PortName=measure  Element=Igd
  In Bus Element1 : Inport  PortName=measure  Element=Igq
  In Bus Element2 : Inport  Port=2  PortName=reactiveControl  Element=Vmd
  In Bus Element4 : Inport  Port=2  PortName=reactiveControl  Element=Vmq
  CurrentLimitingMethod : Subsystem  Variant=on  VariantControlMode=label  VariantControl=Choice  LabelModeActiveChoice=virimp
  Subtract : Sum  Inputs=+-
  Subtract1 : Sum  Inputs=-+
  Out Bus Element : Outport  PortName=currentLimiting  Element=Vmd
  Out Bus Element1 : Outport  PortName=currentLimiting  Element=Vmq
  Out Bus Element2 : Outport  PortName=currentLimiting  Element=Idmax
  Out Bus Element3 : Outport  PortName=currentLimiting  Element=Iqmax
  wires:
  In Bus Element2/1 -> Subtract/1
  In Bus Element1/1 -> CurrentLimitingMethod/2(Igq)
  In Bus Element4/1 -> Subtract1/2
  Subtract/1 -> Out Bus Element/1
  Subtract1/1 -> Out Bus Element1/1
  CurrentLimitingMethod/4(Iqmax) -> Out Bus Element3/1
  In Bus Element/1 -> CurrentLimitingMethod/1(Igd)  "Q"
  CurrentLimitingMethod/3(Idmax) -> Out Bus Element2/1
  CurrentLimitingMethod/1(delVd) -> Subtract/2
  CurrentLimitingMethod/2(delVq) -> Subtract1/1

== system IndustrialMicrogrid/MG1 Primary Substation/BESS and Controller/BESS/Grid-Forming Converter Control/Grid Voltage Reactive Power Support ==
  In Bus Element1 : Inport  PortName=measure  Element=Vgd
  In Bus Element3 : Inport  PortName=measure  Element=Vgq
  In Bus Element2 : Inport  PortName=measure  Element=Igd
  In Bus Element4 : Inport  PortName=measure  Element=Igq
  PrefInput : Inport  Port=2
  QrefInput : Inport  Port=3
  Modifying Active Power Reference : Subsystem
  Modifying Reactive Power Reference : Subsystem
  Pref : Outport
  Qref : Outport  Port=2
  wires:
  Modifying Active Power Reference/1(Pref) -> Modifying Reactive Power Reference/4(Pref)
  PrefInput/1 -> Modifying Active Power Reference/1(PrefInput)
  In Bus Element2/1 -> Modifying Active Power Reference/3(Igd)
  In Bus Element4/1 -> Modifying Active Power Reference/4(Igq)
  In Bus Element1/1 -> Modifying Reactive Power Reference/1(Vgd), Modifying Active Power Reference/2(Vd)
  In Bus Element3/1 -> Modifying Reactive Power Reference/2(Vgq)
  QrefInput/1 -> Modifying Reactive Power Reference/3(Qref)
  Modifying Reactive Power Reference/1(PrefNew) -> Pref/1
  Modifying Reactive Power Reference/2(QrefNew) -> Qref/1

== system IndustrialMicrogrid/MG1 Primary Substation/BESS and Controller/BESS/Grid-Forming Converter Control/Measurement ==
  Vgabcc : Inport
  Igabc : Inport  Port=2
  Angle : Inport  Port=3
  Frequency Measurement : Subsystem
  Gain1 : Gain  Gain=1/power
  Gain2 : Gain  Gain=1/power
  Gain3 : Gain  Gain=1/(girdLineVoltage*sqrt(2/3))
  Gain4 : Gain  Gain=1/(girdLineVoltage*sqrt(2/3))
  Gain5 : Gain  Gain=1/(power/(sqrt(3)*girdLineVoltage)*sqrt(2))
  Gain6 : Gain  Gain=1/(power/(sqrt(3)*girdLineVoltage)*sqrt(2))
  Power Measurement (Three-Phase) : eePowerMeasurement/Power Measurement (Three-Phase)  LabelModeActiveChoice=Discrete  F=powerFreq  K=[1]  Seq=Positive  Ts=measSampleTime
  abc2dq : Subsystem
  Out Bus Element : Outport  PortName=measure  Element=P
  Out Bus Element1 : Outport  PortName=measure  Element=Q
  Out Bus Element2 : Outport  PortName=measure  Element=Vgd
  Out Bus Element3 : Outport  PortName=measure  Element=Vgq
  Out Bus Element4 : Outport  PortName=measure  Element=Igd
  Out Bus Element5 : Outport  PortName=measure  Element=Igq
  Out Bus Element6 : Outport  PortName=measure  Element=fgrid
  Pmeas : Outport  Port=2
  Qmeas : Outport  Port=3
  fmeas : Outport  Port=4
  wires:
  Vgabcc/1 -> abc2dq/3(Vgabc), Frequency Measurement/1(Vabc), Power Measurement (Three-Phase)/1  "Vabc"
  Angle/1 -> abc2dq/2(Angle)
  Power Measurement (Three-Phase)/1 -> Gain2/1
  Igabc/1 -> abc2dq/1(Igabc), Power Measurement (Three-Phase)/2  "Iabc"
  Power Measurement (Three-Phase)/2 -> Gain1/1
  Gain2/1 -> Pmeas/1, Out Bus Element/1  "Pmeas"
  Gain1/1 -> Qmeas/1, Out Bus Element1/1  "Qmeas"
  abc2dq/1(Vgd) -> Gain4/1
  abc2dq/2(Vgq) -> Gain3/1
  abc2dq/3(Igd) -> Gain5/1
  abc2dq/4(Igq) -> Gain6/1
  Gain3/1 -> Out Bus Element3/1  "Vgq"
  Gain4/1 -> Out Bus Element2/1  "Vgd"
  Gain5/1 -> Out Bus Element4/1  "Igd"
  Gain6/1 -> Out Bus Element5/1  "Igq"
  Frequency Measurement/1(freq) -> Out Bus Element6/1, fmeas/1

== system IndustrialMicrogrid/MG1 Primary Substation/BESS and Controller/BESS/Grid-Forming Converter Control/Power Control ==
  note: Reactive Power Control
  note: Active Power Control
  In Bus Element2 : Inport  PortName=measure  Element=P
  In Bus Element1 : Inport  PortName=measure  Element=fgrid
  BusElementIn : Inport  PortName=measure  Element=Vgd
  BusElementIn2 : Inport  PortName=measure  Element=Q
  Pref : Inport  Port=2
  Qref : Inport  Port=3
  Vref : Inport  Port=4
  Fref : Inport  Port=5
  CntrlFlag : Inport  Port=6
  ActivePowerControl : Subsystem  Variant=on  VariantControlMode=label  VariantControl=Choice  LabelModeActiveChoice=vsm
  ReactiveControl : Subsystem
  Scope : Scope
  Out Bus Element : Outport  PortName=reactiveControl  Element=Vmd
  Out Bus Element1 : Outport  PortName=reactiveControl  Element=Vmq
  Out Bus Element6 : Outport  Port=2  PortName=activeControl  Element=angle
  Out Bus Element4 : Outport  Port=2  PortName=activeControl  Element=w
  angle : Outport  Port=3
  wires:
  ActivePowerControl/2(w) -> Out Bus Element4/1
  ActivePowerControl/1(Theta) -> angle/1, Out Bus Element6/1
  ReactiveControl/1(Vmd) -> Out Bus Element/1
  ReactiveControl/2(Vmq) -> Out Bus Element1/1
  Pref/1 -> ActivePowerControl/1(Pref)  "Q"
  Qref/1 -> ReactiveControl/2(Qref)  "Q"
  In Bus Element2/1 -> ActivePowerControl/2(Pmeas)
  In Bus Element1/1 -> ActivePowerControl/5(fgrid)
  Fref/1 -> ActivePowerControl/3(fref)
  CntrlFlag/1 -> [Cntrlflag]
  [Cntrlflag] -> ActivePowerControl/4(cntrlflag)
  Vref/1 -> ReactiveControl/5(Vref)
  [Cntrlflag] -> ReactiveControl/1(CntrlFlag)
  BusElementIn/1 -> Scope/1, ReactiveControl/4(Vgdmeas)
  BusElementIn2/1 -> ReactiveControl/3(Qmeas)

== system IndustrialMicrogrid/MG1 Primary Substation/BESS and Controller/BESS/Grid-Forming Converter Control/VoltageCurrentControl ==
  In Bus Element2 : Inport  PortName=measure  Element=Vgd
  In Bus Element3 : Inport  PortName=measure  Element=Vgq
  In Bus Element4 : Inport  PortName=measure  Element=Igd
  In Bus Element5 : Inport  PortName=measure  Element=Igq
  In Bus Element : Inport  Port=2  PortName=currentLimiting  Element=Vmd
  In Bus Element1 : Inport  Port=2  PortName=currentLimiting  Element=Vmq
  In Bus Element6 : Inport  Port=2  PortName=currentLimiting  Element=Idmax
  In Bus Element7 : Inport  Port=2  PortName=currentLimiting  Element=Iqmax
  Bus Element In6 : Inport  Port=3  PortName=activeControl  Element=w
  Bus Element In1 : Inport  Port=3  PortName=activeControl  Element=angle
  BlackStart : Inport  Port=4
  Controller : Subsystem
      settings: PortSchema="{\"entries\":[{\"content\":{\"sides\":[{\"content\":{\"connectorIds\":[\"In1\",\"In2\",\"In3\",\"In4\",\"In5\",\"In6\",\"In7\",\"In8\",\"In9\"]},\"type\":\"ConnectorPlacement.EquallySpacedRectSide\",\"uuid\":\"29d30ab3-0ae0-4ae6-aaee-46c6f5faca9c\"},{\"content\":{\"connectorIds\":[\"Out1\",\"Out2\"],\"side\":\"RIGHT\"},\"type\":\"ConnectorPlacement.EquallySpacedRectSide\",\"uuid\":\"4918c3a7-9f8f-4af5-ac25-a0a0710917b2\"},{\"content\":{\"connectorIds\":[\"In10\"],\"side\":\"TOP\"},\"type\":\"ConnectorPlacement.EquallySpacedRectSide\",\"uuid\":\"c6ee8000-0a39-46c2-b8e8-8b73a56a82d9\"}]},\"type\":\"ConnectorPlacement.EquallySpacedConnector\",\"uuid\":\"193e0bc8-3764-41d1-9278-3938c4a9e9f5\"}],\"packageUris\":[\"http://schema.mathworks.com/mf0/Connector/R2020b\"],\"version\":\"1.0\"}"
  Modulation Signal : Subsystem
  mabc : Outport
  wires:
  Controller/2(Vq) -> Modulation Signal/2(Vq)
  Modulation Signal/1(mabc) -> mabc/1
  Controller/1(Vd) -> Modulation Signal/1(Vd)
  In Bus Element4/1 -> Controller/6(Id)
  In Bus Element5/1 -> Controller/7(Iq)
  In Bus Element6/1 -> Controller/8(Idmax)
  In Bus Element7/1 -> Controller/9(Iqmax)
  In Bus Element2/1 -> Controller/4(Vsd)
  In Bus Element3/1 -> Controller/5(Vsq)
  Bus Element In6/1 -> Controller/1(Angfreq)
  In Bus Element/1 -> Controller/2(Vgdref)
  In Bus Element1/1 -> Controller/3(Vgqref)
  Bus Element In1/1 -> Modulation Signal/3(Angle)
  BlackStart/1 -> Controller/10(BlackStart1)

== system IndustrialMicrogrid/MG1 Primary Substation/Microgrid Controller/Black Start/If Action Subsystem/Subsystem ==
  Constant2 : Constant  DisableCoverage=on  Value=-(Controller1BlackStart+Controller1BlackStartDelay)  OutDataTypeStr=Inherit: Inherit via back propagation  SampleTime=Ts
  Digital Clock : DigitalClock  SampleTime=Ts
  Output : Sum  Inputs=|++  InputSameDT=on  SaturateOnIntegerOverflow=on  OutDataTypeStr=Inherit: Same as first input
  Product : Product  DisableCoverage=on  InputSameDT=on  SaturateOnIntegerOverflow=on  OutDataTypeStr=Inherit: Same as first input
  Saturation : Saturate  UpperLimit=Controller1BlackStartVoltageLevel1  LowerLimit=0
  Step : Step  DisableCoverage=on  Time=Controller1BlackStart+Controller1BlackStartDelay  OutDataTypeStr=fixdt('double', 'DataTypeOverride', 'Off')  SampleTime=Ts
  Out1 : Outport
  wires:
  Step/1 -> Product/1
  Output/1 -> Saturation/1
  Product/1 -> Output/1
  Saturation/1 -> Out1/1
  Constant2/1 -> Output/2
  Digital Clock/1 -> Product/2

== system IndustrialMicrogrid/MG1 Primary Substation/Microgrid Controller/Black Start/If Action Subsystem/Subsystem1 ==
  Constant2 : Constant  DisableCoverage=on  Value=-(Controller1BlackStart+Controller1BlackStartDelay+Controller1BlackStartDelayLevel2)  OutDataTypeStr=Inherit: Inherit via back propagation  SampleTime=Ts
  Digital Clock : DigitalClock  SampleTime=Ts
  Output : Sum  Inputs=|++  InputSameDT=on  SaturateOnIntegerOverflow=on  OutDataTypeStr=Inherit: Same as first input
  Product : Product  DisableCoverage=on  InputSameDT=on  SaturateOnIntegerOverflow=on  OutDataTypeStr=Inherit: Same as first input
  Saturation : Saturate  UpperLimit=Controller1BlackStartVoltageLevel2  LowerLimit=0
  Step : Step  DisableCoverage=on  Time=Controller1BlackStart+Controller1BlackStartDelay+Controller1BlackStartDelayLevel2  OutDataTypeStr=fixdt('double', 'DataTypeOverride', 'Off')  SampleTime=Ts
  Out1 : Outport
  wires:
  Digital Clock/1 -> Product/2
  Constant2/1 -> Output/2
  Saturation/1 -> Out1/1
  Product/1 -> Output/1
  Output/1 -> Saturation/1
  Step/1 -> Product/1

== system IndustrialMicrogrid/MG1 Primary Substation/Microgrid Controller/Black Start/If Action Subsystem/Subsystem2 ==
  Constant2 : Constant  DisableCoverage=on  Value=-(Controller1BlackStart+Controller1BlackStartDelay+Controller1BlackStartDelayLevel2+Controller1BlackStartDelayLevel3)  OutDataTypeStr=Inherit: Inherit via back propagation  SampleTime=Ts
  Digital Clock : DigitalClock  SampleTime=Ts
  Output : Sum  Inputs=|++  InputSameDT=on  SaturateOnIntegerOverflow=on  OutDataTypeStr=Inherit: Same as first input
  Product : Product  DisableCoverage=on  InputSameDT=on  SaturateOnIntegerOverflow=on  OutDataTypeStr=Inherit: Same as first input
  Saturation : Saturate  UpperLimit=Controller1BlackStartVoltageLevel3  LowerLimit=0
  Step : Step  DisableCoverage=on  Time=Controller1BlackStart+Controller1BlackStartDelay+Controller1BlackStartDelayLevel2+Controller1BlackStartDelayLevel3  OutDataTypeStr=fixdt('double', 'DataTypeOverride', 'Off')  SampleTime=Ts
  Out1 : Outport
  wires:
  Step/1 -> Product/1
  Output/1 -> Saturation/1
  Product/1 -> Output/1
  Saturation/1 -> Out1/1
  Constant2/1 -> Output/2
  Digital Clock/1 -> Product/2

== system IndustrialMicrogrid/MG1 Primary Substation/Microgrid Controller/PLL/PLL/Subsystem ==
  In : Inport
  Bias : Bias  Bias=180  SaturateOnIntegerOverflow=off
  Bias1 : Bias  Bias=-180  SaturateOnIntegerOverflow=off
  Constant : Constant  Value=grid.frequency
  Constant1 : Constant  Value=360
  Data Type Conversion Inherited : simulink/Signal Attributes/Data Type Conversion Inherited  ConvertRealWorld=Real World Value  DoSatur=off
  Digital Clock : DigitalClock  SampleTime=Ts
  Mod : Math  Operator=mod
  Product : Product
  Sum : Sum  Inputs=+-  OutDataTypeStr=Inherit: Same as first input
  gain : Gain  Gain=2*pi
  rad2deg : Gain  Gain=180/pi
  Out : Outport
  wires:
  Data Type Conversion Inherited/1 -> Mod/2
  Sum/1 -> rad2deg/1
  rad2deg/1 -> Bias/1, Data Type Conversion Inherited/1
  Constant1/1 -> Data Type Conversion Inherited/2
  Digital Clock/1 -> Product/2
  Mod/1 -> Bias1/1
  Bias/1 -> Mod/1
  Constant/1 -> gain/1
  gain/1 -> Product/1
  In/1 -> Sum/1
  Product/1 -> Sum/2
  Bias1/1 -> Out/1

== system IndustrialMicrogrid/MG1 Primary Substation/Microgrid Controller/PLL/PLL1/Subsystem ==
  In : Inport
  Bias : Bias  Bias=180  SaturateOnIntegerOverflow=off
  Bias1 : Bias  Bias=-180  SaturateOnIntegerOverflow=off
  Constant : Constant  Value=grid.frequency
  Constant1 : Constant  Value=360
  Data Type Conversion Inherited : simulink/Signal Attributes/Data Type Conversion Inherited  ConvertRealWorld=Real World Value  DoSatur=off
  Digital Clock : DigitalClock  SampleTime=Ts
  Mod : Math  Operator=mod
  Product : Product
  Sum : Sum  Inputs=+-  OutDataTypeStr=Inherit: Same as first input
  gain : Gain  Gain=2*pi
  rad2deg : Gain  Gain=180/pi
  Out : Outport
  wires:
  Bias1/1 -> Out/1
  Product/1 -> Sum/2
  In/1 -> Sum/1
  gain/1 -> Product/1
  Constant/1 -> gain/1
  Bias/1 -> Mod/1
  Mod/1 -> Bias1/1
  Digital Clock/1 -> Product/2
  Constant1/1 -> Data Type Conversion Inherited/2
  rad2deg/1 -> Data Type Conversion Inherited/1, Bias/1
  Sum/1 -> rad2deg/1
  Data Type Conversion Inherited/1 -> Mod/2

== system IndustrialMicrogrid/MG1 Primary Substation/Microgrid Controller/Planned Island/Control for Zero Powerflow/Planned Island Time Delay ==
  In1 : Inport
  In2 : Inport  Port=2
  Cast To Double : DataTypeConversion  OutDataTypeStr=double  SaturateOnIntegerOverflow=off  RndMeth=Floor
  Constant3 : Constant  Value=0
  Delay1 : Delay  DelayLength=500  SampleTime=Ts
  Delay2 : Delay  DelayLength=PlannedIslandDelay  InitialCondition=0  SampleTime=Ts*5
  Monostable Flip-Flop : eeGeneralControl/Monostable Flip-Flop  VariantControl=Variant1  LabelModeActiveChoice=Discrete  ChangeType=Rising edge  x0=0  Td=100  Ts=Ts
      settings: LibrarySourceBlock=ee_sl_lib/General Control/Monostable Flip-Flop
  Switch : Switch  Criteria=u2 > Threshold  Threshold=0.5  SaturateOnIntegerOverflow=off  InputSameDT=off
  MGController : Outport
  wires:
  In2/1 -> Delay1/1
  In1/1 -> Switch/1
  Monostable Flip-Flop/1 -> Cast To Double/1
  Delay2/1 -> MGController/1
  Delay1/1 -> Switch/2
  Constant3/1 -> Switch/3
  Cast To Double/1 -> Delay2/1
  Switch/1 -> Monostable Flip-Flop/1

== system IndustrialMicrogrid/MG1 Primary Substation/Microgrid Controller/Planned Island/Control for Zero Powerflow/Subsystem ==
  AVTIVE POWER ERROR : Inport
  AND : Logic  IconShape=distinctive  AllPortsSameDT=off  OutDataTypeStr=boolean
  Abs : Abs  SaturateOnIntegerOverflow=off
  Constant : Constant  Value=ZeroActivePowerThreshold  SampleTime=-1
  Delay : Delay  DelayLength=1000  SampleTime=Ts
  Relational Operator : RelationalOperator  Operator=<=  OutDataTypeStr=boolean  RndMeth=Simplest  InputSameDT=off
  Out1 : Outport
  wires:
  Delay/1 -> AND/2
  Constant/1 -> Relational Operator/2
  Relational Operator/1 -> AND/1, Delay/1
  AND/1 -> Out1/1
  AVTIVE POWER ERROR/1 -> Abs/1
  Abs/1 -> Relational Operator/1

== system IndustrialMicrogrid/MG1 Primary Substation/Microgrid Controller/Planned Island/Control for Zero Powerflow/Subsystem1 ==
  REACTIVEPOWER ERROR : Inport
  AND : Logic  IconShape=distinctive  AllPortsSameDT=off  OutDataTypeStr=boolean
  Abs : Abs  SaturateOnIntegerOverflow=off
  Constant2 : Constant  Value=ZeroReactivePowerThreshold
  Delay : Delay  DelayLength=1000  SampleTime=Ts
  Relational Operator2 : RelationalOperator  Operator=<=  OutDataTypeStr=boolean  RndMeth=Simplest  InputSameDT=off
  Out1 : Outport
  wires:
  Delay/1 -> AND/2
  REACTIVEPOWER ERROR/1 -> Abs/1
  Relational Operator2/1 -> Delay/1, AND/1
  Constant2/1 -> Relational Operator2/2
  AND/1 -> Out1/1
  Abs/1 -> Relational Operator2/1

== system IndustrialMicrogrid/MG1 Primary Substation/Microgrid Controller/Resynchronization/Frequency and voltage matching/Resynchronization Time Delay ==
  In1 : Inport
  In2 : Inport  Port=2
  Cast To Double : DataTypeConversion  OutDataTypeStr=double  SaturateOnIntegerOverflow=off  RndMeth=Floor
  Constant3 : Constant  Value=0
  Delay1 : Delay  DelayLength=500  SampleTime=Ts
  Delay2 : Delay  DelayLength=ResynchDelay  InitialCondition=0  SampleTime=Ts*5
  Monostable Flip-Flop : eeGeneralControl/Monostable Flip-Flop  VariantControl=Variant1  LabelModeActiveChoice=Discrete  ChangeType=Rising edge  x0=0  Td=100  Ts=Ts
      settings: LibrarySourceBlock=ee_sl_lib/General Control/Monostable Flip-Flop
  Switch : Switch  Criteria=u2 > Threshold  Threshold=0.5  SaturateOnIntegerOverflow=off  InputSameDT=off
  MGController : Outport
  wires:
  Switch/1 -> Monostable Flip-Flop/1
  Cast To Double/1 -> Delay2/1
  Constant3/1 -> Switch/3
  Delay1/1 -> Switch/2
  Delay2/1 -> MGController/1
  Monostable Flip-Flop/1 -> Cast To Double/1
  In1/1 -> Switch/1
  In2/1 -> Delay1/1

== system IndustrialMicrogrid/MG1 Primary Substation/Microgrid Controller/Resynchronization/Frequency and voltage matching/Subsystem ==
  FREQUENCY ERROR : Inport
  AND : Logic  IconShape=distinctive  AllPortsSameDT=off  OutDataTypeStr=boolean
  Abs : Abs  SaturateOnIntegerOverflow=off
  Constant : Constant  Value=FrequencyThreshold  SampleTime=-1
  Delay : Delay  DelayLength=1000  SampleTime=Ts
  Relational Operator : RelationalOperator  Operator=<=  OutDataTypeStr=boolean  RndMeth=Simplest  InputSameDT=off
  Out1 : Outport
  wires:
  Delay/1 -> AND/2
  Constant/1 -> Relational Operator/2
  Relational Operator/1 -> AND/1, Delay/1
  AND/1 -> Out1/1
  FREQUENCY ERROR/1 -> Abs/1
  Abs/1 -> Relational Operator/1

== system IndustrialMicrogrid/MG1 Primary Substation/Microgrid Controller/Resynchronization/Frequency and voltage matching/Subsystem1 ==
  ANGLE ERROR : Inport
  AND : Logic  IconShape=distinctive  AllPortsSameDT=off  OutDataTypeStr=boolean
  Abs : Abs  SaturateOnIntegerOverflow=off
  Constant1 : Constant  Value=AngleThreshold
  Delay : Delay  DelayLength=1000  SampleTime=Ts
  Relational Operator : RelationalOperator  Operator=<=  OutDataTypeStr=boolean  RndMeth=Simplest  InputSameDT=off
  Out1 : Outport
  wires:
  ANGLE ERROR/1 -> Abs/1
  AND/1 -> Out1/1
  Relational Operator/1 -> Delay/1, AND/1
  Constant1/1 -> Relational Operator/2
  Delay/1 -> AND/2
  Abs/1 -> Relational Operator/1

== system IndustrialMicrogrid/MG1 Primary Substation/Microgrid Controller/Resynchronization/Frequency and voltage matching/Subsystem2 ==
  VOLTAGE ERROR : Inport
  AND : Logic  IconShape=distinctive  AllPortsSameDT=off  OutDataTypeStr=boolean
  Abs : Abs  SaturateOnIntegerOverflow=off
  Constant2 : Constant  Value=VoltageThreshold
  Delay : Delay  DelayLength=1000  SampleTime=Ts
  Relational Operator : RelationalOperator  Operator=<=  OutDataTypeStr=boolean  RndMeth=Simplest  InputSameDT=off
  Out1 : Outport
  wires:
  Delay/1 -> AND/2
  Constant2/1 -> Relational Operator/2
  Relational Operator/1 -> AND/1, Delay/1
  AND/1 -> Out1/1
  VOLTAGE ERROR/1 -> Abs/1
  Abs/1 -> Relational Operator/1

== system IndustrialMicrogrid/MG1 Primary Substation/Microgrid Controller/Resynchronization/Frequency and voltage matching/Synch Voltage ==
  MicrogridController : Inport
  ControlRoom : Inport  Port=2
  u : Inport  Port=3
  Resynch : Inport  Port=4
  Gain1 : Gain  Gain=microgrid.KDroop
  Logical Operator1 : Logic  Operator=NOT  AllPortsSameDT=off  OutDataTypeStr=boolean
  Low-Pass Filter (Discrete or Continuous) : eeGeneralControl/Low-Pass Filter (Discrete or Continuous)  K=1  T=0.08  B=inf  A=-inf  init_option=Specify as parameter  x0=0  Ts=5*Ts
  Sample and Hold : spsSampleandHoldLib/Sample and Hold  ic=0  Ts=Ts
  Subsystem2 : Subsystem
  Sum4 : Sum  Inputs=+-
  Out1 : Outport
  wires:
  Low-Pass Filter (Discrete or Continuous)/1 -> Gain1/1
  Resynch/1 -> Logical Operator1/1
  Sample and Hold/1 -> Sum4/1
  Gain1/1 -> Sum4/2
  Logical Operator1/1 -> Sample and Hold/2
  MicrogridController/1 -> Subsystem2/1(MicrogridController)
  Subsystem2/1(Out1) -> Sample and Hold/1
  Sum4/1 -> Out1/1
  ControlRoom/1 -> Subsystem2/2(ControlRoom)
  u/1 -> Low-Pass Filter (Discrete or Continuous)/1
